simulink model "controller_testing"  (R2023b)
settings: Solver=VariableStepAuto  StartTime=0.0  StopTime=20  RelTol=1e-3
libraries: simulink x1
settings Model: Creator=Inver  LastModifiedBy=Inver
settings OptimizationCC: DefaultParameterBehavior=Inlined  UseDivisionForNetSlopeComputation=on  GainParamInheritBuiltInType=on  UseFloatMulNetSlope=on  InlineInvariantSignals=on  PassReuseOutputArgsAs=Individual arguments  ZeroExternalMemoryAtStartup=off  ZeroInternalMemoryAtStartup=off  NoFixptDivByZeroProtection=on  EfficientFloat2IntCast=on  LifeSpan=1  OptimizeBlockOrder=speed  OptimizationPriority=Speed  MultiThreadedLoops=on  EfficientTunableParamExpr=on
settings DebuggingCC: ParameterTunabilityLossMsg=error
settings HardwareCC: ProdBitPerPointer=32  ProdBitPerSizeT=32  ProdBitPerPtrDiffT=32  ProdLargestAtomicInteger=Long  ProdLargestAtomicFloat=Double  ProdWordSize=32  ProdLongLongMode=on  ProdHWDeviceType=ARM Compatible->ARM Cortex-M
settings SFSimCC: SimCustomHeaderCode="#include \"simplex.h\""  SimUserSources=simplex.c  MATLABDynamicMemAlloc=off
settings RTWCC: Description=Embedded Coder  SystemTargetFile=ert.tlc  GenCodeOnly=on  PackageGeneratedCodeAndArtifacts=on  TemplateMakefile=ert_default_tmf  Toolchain=GNU Tools for ARM Embedded Processors  BuildConfiguration=Faster Runs  CodeExecutionProfiling=on  CodeProfilingInstrumentation=detailed
settings CodeAppCC: ForceParamTrailComments=on  IgnoreCustomStorageClasses=off  OperatorAnnotations=on  SimulinkDataObjDesc=on  SFDataObjDesc=on  CustomSymbolStrGlobalVar=rt$N$M  CustomSymbolStrType=$N$M  CustomSymbolStrFcn=$N$M$F  CustomSymbolStrMacro=$N$M  InsertBlockDesc=on
settings ERTTargetCC: TargetLangStandard=C99 (ISO)  GenerateSampleERTMain=on  IncludeMdlTerminateFcn=off  CombineSignalStateStructs=on  CodeInterfacePackaging=Reusable function  SupportComplex=off  SupportNonInlinedSFcns=on  InlinedParameterPlacement=NonHierarchical  RootIOFormat=Structure reference  ERTCustomFileTemplate=example_file_process.tlc  GlobalDataDefinition=InSeparateSourceFile  DataDefinitionFile=data.c  GlobalDataReference=InSeparateHeaderFile  ERTFilePackagingFormat=CompactWithDataFile  DataReferenceFile=data.h

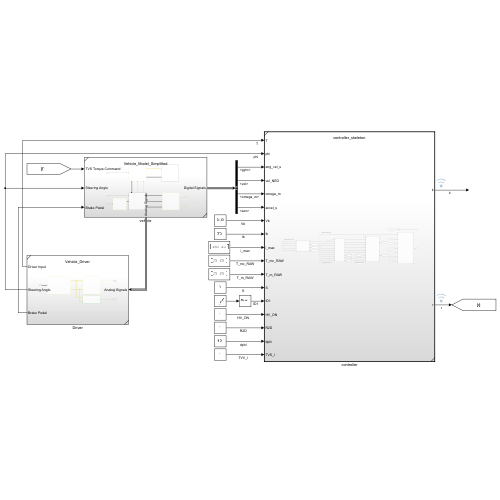
[thumbnail: Simulink's stored preview of the top-level diagram]
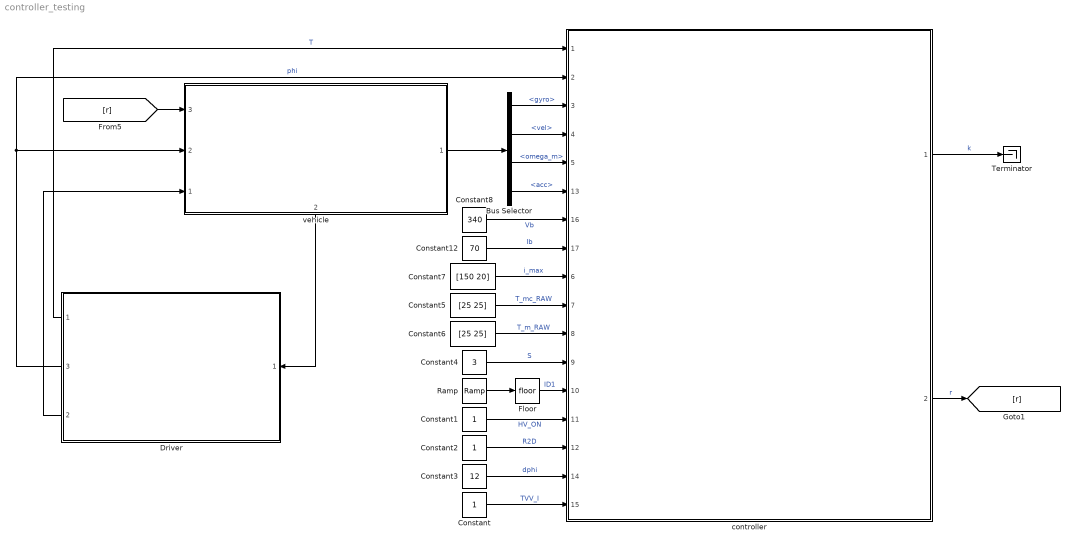
== system controller_testing ==
  Bus Selector : BusSelector  OutputSignals=Navigation Sensors.gyro,Navigation Sensors.vel,Corner Dynamics Sensors.omega_m,Navigation Sensors.acc
  Constant : Constant
  Constant1 : Constant
  Constant12 : Constant  Value=70
  Constant2 : Constant
  Constant3 : Constant  Value=12
  Constant4 : Constant  Value=3
  Constant5 : Constant  Value=[25 25]
  Constant6 : Constant  Value=[25 25]
  Constant7 : Constant  Value=[150 20]
  Constant8 : Constant  Value=340
  Driver : Subsystem  ReferencedSubsystem=Vehicle_Driver
      settings: PortSchema="{\"entries\":[{\"content\":{\"sides\":[{\"content\":{\"connectorIds\":[\"Out1\",\"Out3\",\"Out2\"]},\"type\":\"ConnectorPlacement.EquallySpacedRectSide\",\"uuid\":\"c8f3518c-48c1-48e6-bf49-b5946aebc156\"},{\"content\":{\"connectorIds\":[\"In1\"],\"side\":\"RIGHT\"},\"type\":\"ConnectorPlacement.EquallySpacedRectSide\",\"uuid\":\"d1ff2ecd-3804-4616-be8b-c7741816ffed\"},{\"content\":{\"side\":\"TOP\"},\"type\":\"ConnectorPlacement.EquallySpacedRectSide\",\"uuid\":\"0d6b10aa-d497-4cfd-b6f3-3ffc80b2cc8c\"}]},\"type\":\"ConnectorPlacement.EquallySpacedConnector\",\"uuid\":\"8189dedf-d1b1-471b-a005-48bc7d1d6f32\"}],\"packageUris\":[\"http://schema.mathworks.com/mf0/Connector/R2020b\"],\"version\":\"1.0\"}"
  Floor : Rounding
  Ramp : simulink/Sources/Ramp  slope=50  start=0  InitialOutput=zeros(1,10)
  Terminator : Terminator
  controller : Subsystem  TreatAsAtomicUnit=on  SystemSampleTime=0.02  ReferencedSubsystem=controller_skeleton
      settings: PortSchema="{\"entries\":[{\"content\":{\"sides\":[{\"content\":{\"connectorIds\":[\"In1\",\"In2\",\"In3\",\"In4\",\"In5\",\"In13\",\"In16\",\"In17\",\"In6\",\"In7\",\"In8\",\"In9\",\"In10\",\"In11\",\"In12\",\"In14\",\"In15\"]},\"type\":\"ConnectorPlacement.EquallySpacedRectSide\",\"uuid\":\"0b0347ce-ee5a-4fdf-9414-e1397c326178\"},{\"content\":{\"connectorIds\":[\"Out1\",\"Out2\"],\"side\":\"RIGHT\"},\"type\":\"ConnectorPlacement.EquallySpacedRectSide\",\"uuid\":\"b979d760-a217-4039-ab00-f24be44979f6\"},{\"content\":{\"side\":\"TOP\"},\"type\":\"ConnectorPlacement.EquallySpacedRectSide\",\"uuid\":\"301f12dd-c094-4a8f-a587-0207ca398211\"}]},\"type\":\"ConnectorPlacement.EquallySpacedConnector\",\"uuid\":\"dc35bc61-9462-4200-b13b-340af4020d66\"}],\"packageUris\":[\"http://schema.mathworks.com/mf0/Connector/R2020b\"],\"version\":\"1.0\"}"
  vehicle : Subsystem  ReferencedSubsystem=Vehicle_Model_Simplified
      settings: PortSchema="{\"entries\":[{\"content\":{\"sides\":[{\"content\":{\"connectorIds\":[\"In3\",\"In2\",\"In1\"]},\"type\":\"ConnectorPlacement.EquallySpacedRectSide\",\"uuid\":\"8b7d0458-19e6-4f5f-a2ba-6896bc8547a5\"},{\"content\":{\"connectorIds\":[\"Out1\"],\"side\":\"RIGHT\"},\"type\":\"ConnectorPlacement.EquallySpacedRectSide\",\"uuid\":\"a43880ad-82fe-45ef-8c70-24ac571715de\"},{\"content\":{\"side\":\"TOP\"},\"type\":\"ConnectorPlacement.EquallySpacedRectSide\",\"uuid\":\"66574ddc-a488-4804-99cd-be4e95fcc69f\"},{\"content\":{\"connectorIds\":[\"Out2\"],\"side\":\"BOTTOM\"},\"type\":\"ConnectorPlacement.EquallySpacedRectSide\",\"uuid\":\"fabe72c8-70b5-4979-b7ad-47d1f12336ef\"}]},\"type\":\"ConnectorPlacement.EquallySpacedConnector\",\"uuid\":\"a0af0009-be5b-43ca-b50b-758f5d04f5dc\"}],\"packageUris\":[\"http://schema.mathworks.com/mf0/Connector/R2020b\"],\"version\":\"1.0\"}"
  wires:
  Constant/1 -> controller/15  "TVV_I"
  Constant3/1 -> controller/14  "dphi"
  Constant2/1 -> controller/12  "R2D"
  Constant1/1 -> controller/11  "HV_ON"
  Constant4/1 -> controller/9  "S"
  Constant5/1 -> controller/7  "T_mc_RAW"
  Constant6/1 -> controller/8  "T_m_RAW"
  Constant7/1 -> controller/6  "i_max"
  Ramp/1 -> Floor/1
  Floor/1 -> controller/10  "ID1"
  Constant8/1 -> controller/16  "Vb"
  controller/1 -> Terminator/1  "k"
  Driver/1 -> controller/1  "T"
  Driver/3 -> controller/2, vehicle/2  "phi"
  Driver/2 -> vehicle/1
  vehicle/1 -> Bus Selector/1
  Bus Selector/1 -> controller/3  "<gyro>"
  Bus Selector/2 -> controller/4  "<vel>"
  Bus Selector/3 -> controller/5  "<omega_m>"
  Bus Selector/4 -> controller/13  "<acc>"
  Constant12/1 -> controller/17  "Ib"
  controller/2 -> [r]  "r"
  [r] -> vehicle/3
  vehicle/2 -> Driver/1
